simulink model "eCS_Old_Algo_And_Tests"  (R2015b)
settings: Solver=VariableStepAuto  StartTime=0.0  StopTime=10.0  RelTol=1e-3
values from neighbouring files (symbols this model uses):
  pulsetype = 2    [Parameter_eCS_Algo.m]    (also in run_simulation.m = j; run_simulation_ActiveX.m = j)
  rotation = 0    [Parameter_eCS_Algo.m]
  SubPulseType = 1    [Parameter_eCS_Algo.m]
undefined symbols (not defined in the file or in its folder): ddv, DiscIntNeverNeededParam, ECE_45_ax, ECE_45_ay, ECE_45_time, gmw_roada_x__m_s__, gmw_roada_y__m_s__, gmw_roadtime_2kHz, Heiko_AY, Heiko_AY_time, Meldorf_HindenburgstraAcceleration_x__m_s_2_, Meldorf_HindenburgstraAcceleration_y__m_s_2_, Meldorf_HindenburgstraTime__s_, pulse_FF27, pulse_MPDB, pulse_ODB40, pulse_ODB64, pulse_USNCAP, pulsetime_FF27, pulsetime_MPDB, pulsetime_ODB40, pulsetime_ODB64, pulsetime_USNCAP, VW_416_2kHza_x_2kHz, VW_416_2kHza_y_2kHz, VW_416_2kHztime_2kHz
libraries: tllib x9, simulink x9
(part 3 of 8)

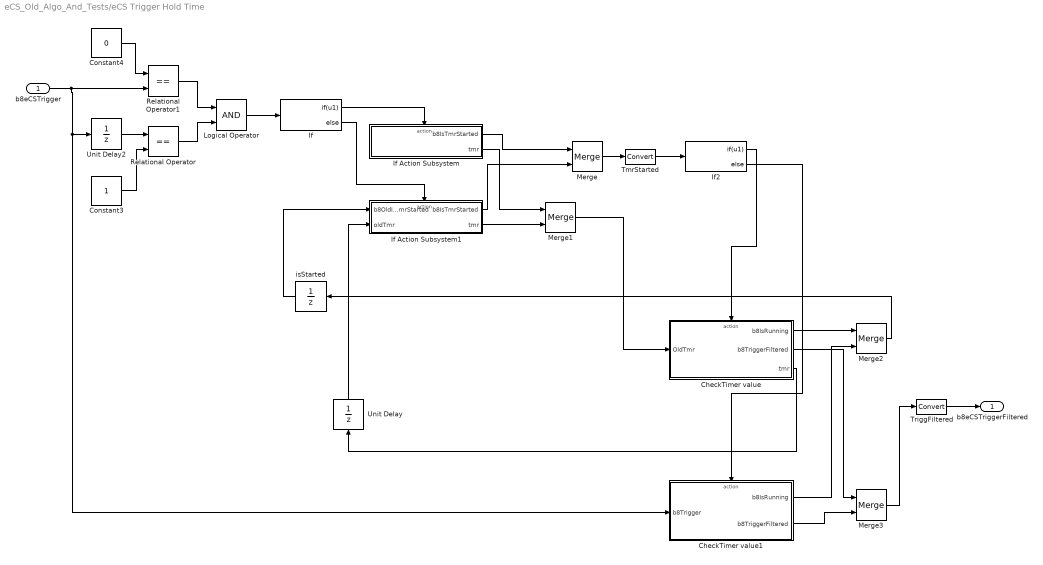
== system eCS_Old_Algo_And_Tests/eCS Trigger Hold Time ==
  b8eCSTrigger : Inport
  CheckTimer value : Subsystem  TreatAsAtomicUnit=on
  CheckTimer value1 : Subsystem  TreatAsAtomicUnit=on
  Constant3 : Constant  mask(TL_Constant){data={'date',738071.59305222228}}
      settings: CopyFcn=if exist('tl_reset_reviewflag') == 2, tl_reset_reviewflag(gcbh); end  DeleteFcn=if exist('delete_tlblock','file')==2,delete_tlblock(gcbh);end  NameChangeFcn=if exist('rename_tlblock','file')==2,rename_tlblock(gcbh);end  OpenFcn=if exist('tl_open_blockdlg','file')==2,tl_open_blockdlg(gcbh);else,open_system(gcbh,'parameter');end
      mask Help: eval(['if exist(''tl_online_help'',''file'') == 2, tl_online_help(''Topic'',''TL_Constant''),else, web([''jar:file:///'',matlabroot,''/help/toolbox/simulink/help.jar!/slref/' lower(get_param(gcbh,'Blocktype')) '.html''], ''-helpbrowser''),end'])
      mask Display: plot([-0.1, 1.05, NaN, -0.1, 1.05],[.01, .01, NaN, .99, .99]);
  Constant4 : Constant  Value=0  mask(TL_Constant){data={'date',738071.59305231483}}
      settings: CopyFcn=if exist('tl_reset_reviewflag') == 2, tl_reset_reviewflag(gcbh); end  DeleteFcn=if exist('delete_tlblock','file')==2,delete_tlblock(gcbh);end  NameChangeFcn=if exist('rename_tlblock','file')==2,rename_tlblock(gcbh);end  OpenFcn=if exist('tl_open_blockdlg','file')==2,tl_open_blockdlg(gcbh);else,open_system(gcbh,'parameter');end
      mask Help: eval(['if exist(''tl_online_help'',''file'') == 2, tl_online_help(''Topic'',''TL_Constant''),else, web([''jar:file:///'',matlabroot,''/help/toolbox/simulink/help.jar!/slref/' lower(get_param(gcbh,'Blocktype')) '.html''], ''-helpbrowser''),end'])
      mask Display: plot([-0.1, 1.05, NaN, -0.1, 1.05],[.01, .01, NaN, .99, .99]);
  If : If  IfExpression=u1
  If Action Subsystem : Subsystem  TreatAsAtomicUnit=on
  If Action Subsystem1 : Subsystem  TreatAsAtomicUnit=on
  If2 : If  IfExpression=u1
  Logical Operator : Logic  AllPortsSameDT=off  OutDataTypeStr=boolean  mask(TL_LogicalOperator){data={'date',738071.59305260412}}
      settings: DeleteFcn=if exist('delete_tlblock','file')==2,delete_tlblock(gcbh);end  NameChangeFcn=if exist('rename_tlblock','file')==2,rename_tlblock(gcbh);end  OpenFcn=if exist('tl_open_blockdlg','file')==2,tl_open_blockdlg(gcbh);else,open_system(gcbh,'parameter');end
      mask Help: eval(['if exist(''tl_online_help'',''file'') == 2, tl_online_help(''Topic'',''TL_LogicalOperator''),else, web([''jar:file:///'',matlabroot,''/help/toolbox/simulink/help.jar!/slref/' lower(get_param(gcbh,'Blocktype')) '.html''], ''-helpbrowser''),end'])
      mask Display: plot([-0.1, 1.05, NaN, -0.1, 1.05],[.01, .01, NaN, .99, .99]);
  Merge : Merge  InitialOutput=0  mask(TL_Merge){data={'date',738071.59305268514}}
      settings: CopyFcn=if exist('tl_reset_reviewflag') == 2, tl_reset_reviewflag(gcbh); end  DeleteFcn=if exist('delete_tlblock','file')==2,delete_tlblock(gcbh);end  NameChangeFcn=if exist('rename_tlblock','file')==2,rename_tlblock(gcbh);end  OpenFcn=if exist('tl_open_blockdlg','file')==2,tl_open_blockdlg(gcbh);else,open_system(gcbh,'parameter');end
      mask Help: eval(['if exist(''tl_online_help'',''file'') == 2, tl_online_help(''Topic'',''TL_Merge''),else, web([''jar:file:///'',matlabroot,''/help/toolbox/simulink/help.jar!/slref/' lower(get_param(gcbh,'Blocktype')) '.html''], ''-helpbrowser''),end'])
      mask Display: plot([-0.1, 1.05, NaN, -0.1, 1.05],[.01, .01, NaN, .99, .99]);
  Merge1 : Merge  InitialOutput=0  mask(TL_Merge){data={'date',738071.59305276617}}
      settings: CopyFcn=if exist('tl_reset_reviewflag') == 2, tl_reset_reviewflag(gcbh); end  DeleteFcn=if exist('delete_tlblock','file')==2,delete_tlblock(gcbh);end  NameChangeFcn=if exist('rename_tlblock','file')==2,rename_tlblock(gcbh);end  OpenFcn=if exist('tl_open_blockdlg','file')==2,tl_open_blockdlg(gcbh);else,open_system(gcbh,'parameter');end
      mask Help: eval(['if exist(''tl_online_help'',''file'') == 2, tl_online_help(''Topic'',''TL_Merge''),else, web([''jar:file:///'',matlabroot,''/help/toolbox/simulink/help.jar!/slref/' lower(get_param(gcbh,'Blocktype')) '.html''], ''-helpbrowser''),end'])
      mask Display: plot([-0.1, 1.05, NaN, -0.1, 1.05],[.01, .01, NaN, .99, .99]);
  Merge2 : Merge  InitialOutput=0  mask(TL_Merge){data={'date',738071.59305284719}}
      settings: CopyFcn=if exist('tl_reset_reviewflag') == 2, tl_reset_reviewflag(gcbh); end  DeleteFcn=if exist('delete_tlblock','file')==2,delete_tlblock(gcbh);end  NameChangeFcn=if exist('rename_tlblock','file')==2,rename_tlblock(gcbh);end  OpenFcn=if exist('tl_open_blockdlg','file')==2,tl_open_blockdlg(gcbh);else,open_system(gcbh,'parameter');end
      mask Help: eval(['if exist(''tl_online_help'',''file'') == 2, tl_online_help(''Topic'',''TL_Merge''),else, web([''jar:file:///'',matlabroot,''/help/toolbox/simulink/help.jar!/slref/' lower(get_param(gcbh,'Blocktype')) '.html''], ''-helpbrowser''),end'])
      mask Display: plot([-0.1, 1.05, NaN, -0.1, 1.05],[.01, .01, NaN, .99, .99]);
  Merge3 : Merge  InitialOutput=0  mask(TL_Merge){data={'date',738071.59305292822}}
      settings: CopyFcn=if exist('tl_reset_reviewflag') == 2, tl_reset_reviewflag(gcbh); end  DeleteFcn=if exist('delete_tlblock','file')==2,delete_tlblock(gcbh);end  NameChangeFcn=if exist('rename_tlblock','file')==2,rename_tlblock(gcbh);end  OpenFcn=if exist('tl_open_blockdlg','file')==2,tl_open_blockdlg(gcbh);else,open_system(gcbh,'parameter');end
      mask Help: eval(['if exist(''tl_online_help'',''file'') == 2, tl_online_help(''Topic'',''TL_Merge''),else, web([''jar:file:///'',matlabroot,''/help/toolbox/simulink/help.jar!/slref/' lower(get_param(gcbh,'Blocktype')) '.html''], ''-helpbrowser''),end'])
      mask Display: plot([-0.1, 1.05, NaN, -0.1, 1.05],[.01, .01, NaN, .99, .99]);
  Relational Operator : RelationalOperator  Operator===  OutDataTypeStr=boolean  mask(TL_RelationalOperator){data={'date',738071.59305300924}}
      settings: DeleteFcn=if exist('delete_tlblock','file')==2,delete_tlblock(gcbh);end  NameChangeFcn=if exist('rename_tlblock','file')==2,rename_tlblock(gcbh);end  OpenFcn=if exist('tl_open_blockdlg','file')==2,tl_open_blockdlg(gcbh);else,open_system(gcbh,'parameter');end
      mask Help: eval(['if exist(''tl_online_help'',''file'') == 2, tl_online_help(''Topic'',''TL_RelationalOperator''),else, web([''jar:file:///'',matlabroot,''/help/toolbox/simulink/help.jar!/slref/' lower(get_param(gcbh,'Blocktype')) '.html''], ''-helpbrowser''),end'])
      mask Display: plot([-0.1, 1.05, NaN, -0.1, 1.05],[.01, .01, NaN, .99, .99]);
  Relational Operator1 : RelationalOperator  Operator===  OutDataTypeStr=boolean  mask(TL_RelationalOperator){data={'date',738071.59305305558}}
      settings: DeleteFcn=if exist('delete_tlblock','file')==2,delete_tlblock(gcbh);end  NameChangeFcn=if exist('rename_tlblock','file')==2,rename_tlblock(gcbh);end  OpenFcn=if exist('tl_open_blockdlg','file')==2,tl_open_blockdlg(gcbh);else,open_system(gcbh,'parameter');end
      mask Help: eval(['if exist(''tl_online_help'',''file'') == 2, tl_online_help(''Topic'',''TL_RelationalOperator''),else, web([''jar:file:///'',matlabroot,''/help/toolbox/simulink/help.jar!/slref/' lower(get_param(gcbh,'Blocktype')) '.html''], ''-helpbrowser''),end'])
      mask Display: plot([-0.1, 1.05, NaN, -0.1, 1.05],[.01, .01, NaN, .99, .99]);
  TmrStarted : DataTypeConversion  mask(TL_Rescaler){data={'output',{'type','Bool'},'date',738071.59305305558}}
      settings: DeleteFcn=if exist('delete_tlblock','file')==2,delete_tlblock(gcbh);end  NameChangeFcn=if exist('rename_tlblock','file')==2,rename_tlblock(gcbh);end  OpenFcn=if exist('tl_open_blockdlg','file')==2,tl_open_blockdlg(gcbh);else,open_system(gcbh,'parameter');end
      mask Help: eval(['if exist(''tl_online_help'',''file'') == 2, tl_online_help(''Topic'',''TL_Rescaler''),else, web([''jar:file:///'',matlabroot,''/help/toolbox/simulink/help.jar!/slref/' lower(get_param(gcbh,'Blocktype')) '.html''], ''-helpbrowser''),end'])
      mask Display: plot([-0.1, 1.05, NaN, -0.1, 1.05],[.01, .01, NaN, .99, .99]);
  TriggFiltered : DataTypeConversion  mask(TL_Rescaler){data={'output',{'type','Bool'},'date',738073.43387922458}}
      settings: DeleteFcn=if exist('delete_tlblock','file')==2,delete_tlblock(gcbh);end  NameChangeFcn=if exist('rename_tlblock','file')==2,rename_tlblock(gcbh);end  OpenFcn=if exist('tl_open_blockdlg','file')==2,tl_open_blockdlg(gcbh);else,open_system(gcbh,'parameter');end
      mask Help: eval(['if exist(''tl_online_help'',''file'') == 2, tl_online_help(''Topic'',''TL_Rescaler''),else, web([''jar:file:///'',matlabroot,''/help/toolbox/simulink/help.jar!/slref/' lower(get_param(gcbh,'Blocktype')) '.html''], ''-helpbrowser''),end'])
      mask Display: plot([-0.1, 1.05, NaN, -0.1, 1.05],[.01, .01, NaN, .99, .99]);
  Unit Delay : UnitDelay  SampleTime=-1  mask(TL_UnitDelay){data={'output',{'type','UInt16'},'state',{'type','UInt16'},'date',738071.59305334487}}
      settings: CopyFcn=if exist('tl_reset_reviewflag') == 2, tl_reset_reviewflag(gcbh); end  DeleteFcn=if exist('delete_tlblock','file')==2,delete_tlblock(gcbh);end  NameChangeFcn=if exist('rename_tlblock','file')==2,rename_tlblock(gcbh);end  OpenFcn=if exist('tl_open_blockdlg','file')==2,tl_open_blockdlg(gcbh);else,open_system(gcbh,'parameter');end
      mask Help: eval(['if exist(''tl_online_help'',''file'') == 2, tl_online_help(''Topic'',''TL_UnitDelay''),else, web([''jar:file:///'',matlabroot,''/help/toolbox/simulink/help.jar!/slref/' lower(get_param(gcbh,'Blocktype')) '.html''], ''-helpbrowser''),end'])
      mask Display: plot([-0.1, 1.05, NaN, -0.1, 1.05],[.01, .01, NaN, .99, .99]);
  Unit Delay2 : UnitDelay  SampleTime=-1  mask(TL_UnitDelay){data={'output',{'type','UInt8'},'state',{'type','UInt8'},'date',738071.59305344906}}
      settings: CopyFcn=if exist('tl_reset_reviewflag') == 2, tl_reset_reviewflag(gcbh); end  DeleteFcn=if exist('delete_tlblock','file')==2,delete_tlblock(gcbh);end  NameChangeFcn=if exist('rename_tlblock','file')==2,rename_tlblock(gcbh);end  OpenFcn=if exist('tl_open_blockdlg','file')==2,tl_open_blockdlg(gcbh);else,open_system(gcbh,'parameter');end
      mask Help: eval(['if exist(''tl_online_help'',''file'') == 2, tl_online_help(''Topic'',''TL_UnitDelay''),else, web([''jar:file:///'',matlabroot,''/help/toolbox/simulink/help.jar!/slref/' lower(get_param(gcbh,'Blocktype')) '.html''], ''-helpbrowser''),end'])
      mask Display: plot([-0.1, 1.05, NaN, -0.1, 1.05],[.01, .01, NaN, .99, .99]);
  isStarted : UnitDelay  SampleTime=-1  mask(TL_UnitDelay){data={'output',{'type','Bool'},'state',{'type','Bool'},'date',738071.59305354161}}
      settings: CopyFcn=if exist('tl_reset_reviewflag') == 2, tl_reset_reviewflag(gcbh); end  DeleteFcn=if exist('delete_tlblock','file')==2,delete_tlblock(gcbh);end  NameChangeFcn=if exist('rename_tlblock','file')==2,rename_tlblock(gcbh);end  OpenFcn=if exist('tl_open_blockdlg','file')==2,tl_open_blockdlg(gcbh);else,open_system(gcbh,'parameter');end
      mask Help: eval(['if exist(''tl_online_help'',''file'') == 2, tl_online_help(''Topic'',''TL_UnitDelay''),else, web([''jar:file:///'',matlabroot,''/help/toolbox/simulink/help.jar!/slref/' lower(get_param(gcbh,'Blocktype')) '.html''], ''-helpbrowser''),end'])
      mask Display: plot([-0.1, 1.05, NaN, -0.1, 1.05],[.01, .01, NaN, .99, .99]);
  b8eCSTriggerFiltered : Outport
  wires:
  TmrStarted/1 -> If2/1
  Merge1/1 -> CheckTimer value/1(OldTmr)
  TriggFiltered/1 -> b8eCSTriggerFiltered/1
  Merge3/1 -> TriggFiltered/1
  CheckTimer value1/1(b8IsRunning) -> Merge2/2
  CheckTimer value/1(b8IsRunning) -> Merge2/1
  Merge2/1 -> isStarted/1
  If2/2 -> CheckTimer value1/Action
  Unit Delay/1 -> If Action Subsystem1/2(oldTmr)
  CheckTimer value/3(tmr) -> Unit Delay/1
  If Action Subsystem1/2(tmr) -> Merge1/2
  If Action Subsystem/2(tmr) -> Merge1/1
  isStarted/1 -> If Action Subsystem1/1(b8OldIsTmrStarted)
  Merge/1 -> TmrStarted/1
  If Action Subsystem1/1(b8IsTmrStarted) -> Merge/2
  If Action Subsystem/1(b8IsTmrStarted) -> Merge/1
  If/2 -> If Action Subsystem1/Action
  Relational Operator/1 -> Logical Operator/2
  Relational Operator1/1 -> Logical Operator/1
  Logical Operator/1 -> If/1
  Constant4/1 -> Relational Operator1/1
  Constant3/1 -> Relational Operator/2
  Unit Delay2/1 -> Relational Operator/1
  b8eCSTrigger/1 -> Unit Delay2/1, CheckTimer value1/1(b8Trigger), Relational Operator1/2
  If2/1 -> CheckTimer value/Action
  If/1 -> If Action Subsystem/Action
  CheckTimer value1/2(b8TriggerFiltered) -> Merge3/2
  CheckTimer value/2(b8TriggerFiltered) -> Merge3/1

== system eCS_Old_Algo_And_Tests/eCS_Algo_in_g ==
  Ax (g) : Inport  PortDimensions=1
  Ay (g) : Inport  Port=2  PortDimensions=1
  Action Port : ActionPort
  Ax dual integrator : Subsystem  TreatAsAtomicUnit=on
  Ay dual integrator : Subsystem  TreatAsAtomicUnit=on
  Crash Acceleration : Subsystem  TreatAsAtomicUnit=on
  Gain : Gain  Gain=ddv('gSecSquareToMM')  mask(TL_Gain){data={'output',{'type','UInt16','lsb',2^-14,'unit','m'},'gain',{'variable','gSecSquareToMM'},'date',737951.40928561345}}
      settings: CopyFcn=if exist('tl_reset_reviewflag') == 2, tl_reset_reviewflag(gcbh); end  DeleteFcn=if exist('delete_tlblock','file')==2,delete_tlblock(gcbh);end  NameChangeFcn=if exist('rename_tlblock','file')==2,rename_tlblock(gcbh);end  OpenFcn=if exist('tl_open_blockdlg','file')==2,tl_open_blockdlg(gcbh);else,open_system(gcbh,'parameter');end
      mask Help: eval(['if exist(''tl_online_help'',''file'') == 2, tl_online_help(''Topic'',''TL_Gain''),else, web([''jar:file:///'',matlabroot,''/help/toolbox/simulink/help.jar!/slref/' lower(get_param(gcbh,'Blocktype')) '.html''], ''-helpbrowser''),end'])
      mask Display: plot([0, .88, 0],[.05, .5, .93]);
  Vector Norm : Subsystem  TreatAsAtomicUnit=on
  eCS Trigger Hold Time : Subsystem  TreatAsAtomicUnit=on
  mergedTrigger : Logic  Operator=OR  AllPortsSameDT=off  OutDataTypeStr=boolean  mask(TL_LogicalOperator){data={'date',737961.51872327551}}
      settings: DeleteFcn=if exist('delete_tlblock','file')==2,delete_tlblock(gcbh);end  NameChangeFcn=if exist('rename_tlblock','file')==2,rename_tlblock(gcbh);end  OpenFcn=if exist('tl_open_blockdlg','file')==2,tl_open_blockdlg(gcbh);else,open_system(gcbh,'parameter');end
      mask Help: eval(['if exist(''tl_online_help'',''file'') == 2, tl_online_help(''Topic'',''TL_LogicalOperator''),else, web([''jar:file:///'',matlabroot,''/help/toolbox/simulink/help.jar!/slref/' lower(get_param(gcbh,'Blocktype')) '.html''], ''-helpbrowser''),end'])
      mask Display: plot([-0.1, 1.05, NaN, -0.1, 1.05],[.01, .01, NaN, .99, .99]);
  s_ball : Outport
  eCSTrigger : Outport  Port=2
  wires:
  Gain/1 -> s_ball/1
  Ay dual integrator/1(Sy (g.s²)) -> Vector Norm/2(Sy)
  Crash Acceleration/1(b8CrashTrigger) -> mergedTrigger/2
  Ax dual integrator/1(Sx (g.s²)) -> Vector Norm/1(Sx)
  Ay (g)/1 -> Ay dual integrator/1(Ay (g)), Crash Acceleration/2(Ay)
  eCS Trigger Hold Time/1(b8eCSTriggerFiltered) -> eCSTrigger/1
  Vector Norm/1(s_ball) -> Gain/1
  Ax (g)/1 -> Crash Acceleration/1(Ax), Ax dual integrator/1(Ax (g))
  Vector Norm/2(b8PositionTrigger) -> mergedTrigger/1
  mergedTrigger/1 -> eCS Trigger Hold Time/1(b8eCSTrigger)

== system eCS_Old_Algo_And_Tests/eCS_Algo_in_g1 ==
  Ax (g) : Inport  PortDimensions=1
  Ay (g) : Inport  Port=2  PortDimensions=1
  Action Port : ActionPort
  Ax dual integrator : Subsystem  TreatAsAtomicUnit=on
  Ay dual integrator : Subsystem  TreatAsAtomicUnit=on
  Crash Acceleration : Subsystem  TreatAsAtomicUnit=on
  Gain : Gain  Gain=ddv('gSecSquareToMM')  mask(TL_Gain){data={'output',{'type','UInt16','lsb',2^-14,'unit','m'},'gain',{'variable','gSecSquareToMM'},'date',737951.40928561345}}
      settings: CopyFcn=if exist('tl_reset_reviewflag') == 2, tl_reset_reviewflag(gcbh); end  DeleteFcn=if exist('delete_tlblock','file')==2,delete_tlblock(gcbh);end  NameChangeFcn=if exist('rename_tlblock','file')==2,rename_tlblock(gcbh);end  OpenFcn=if exist('tl_open_blockdlg','file')==2,tl_open_blockdlg(gcbh);else,open_system(gcbh,'parameter');end
      mask Help: eval(['if exist(''tl_online_help'',''file'') == 2, tl_online_help(''Topic'',''TL_Gain''),else, web([''jar:file:///'',matlabroot,''/help/toolbox/simulink/help.jar!/slref/' lower(get_param(gcbh,'Blocktype')) '.html''], ''-helpbrowser''),end'])
      mask Display: plot([0, .88, 0],[.05, .5, .93]);
  Vector Norm : Subsystem  TreatAsAtomicUnit=on
  eCS Trigger Hold Time : Subsystem  TreatAsAtomicUnit=on
  mergedTrigger : Logic  Operator=OR  AllPortsSameDT=off  OutDataTypeStr=boolean  mask(TL_LogicalOperator){data={'date',737961.51872327551}}
      settings: DeleteFcn=if exist('delete_tlblock','file')==2,delete_tlblock(gcbh);end  NameChangeFcn=if exist('rename_tlblock','file')==2,rename_tlblock(gcbh);end  OpenFcn=if exist('tl_open_blockdlg','file')==2,tl_open_blockdlg(gcbh);else,open_system(gcbh,'parameter');end
      mask Help: eval(['if exist(''tl_online_help'',''file'') == 2, tl_online_help(''Topic'',''TL_LogicalOperator''),else, web([''jar:file:///'',matlabroot,''/help/toolbox/simulink/help.jar!/slref/' lower(get_param(gcbh,'Blocktype')) '.html''], ''-helpbrowser''),end'])
      mask Display: plot([-0.1, 1.05, NaN, -0.1, 1.05],[.01, .01, NaN, .99, .99]);
  s_ball : Outport
  eCSTrigger : Outport  Port=2
  wires:
  Gain/1 -> s_ball/1
  Ay dual integrator/1(Sy (g.s²)) -> Vector Norm/2(Sy)
  Crash Acceleration/1(b8CrashTrigger) -> mergedTrigger/2
  Ax dual integrator/1(Sx (g.s²)) -> Vector Norm/1(Sx)
  Ay (g)/1 -> Ay dual integrator/1(Ay (g)), Crash Acceleration/2(Ay)
  eCS Trigger Hold Time/1(b8eCSTriggerFiltered) -> eCSTrigger/1
  Vector Norm/1(s_ball) -> Gain/1
  Ax (g)/1 -> Crash Acceleration/1(Ax), Ax dual integrator/1(Ax (g))
  Vector Norm/2(b8PositionTrigger) -> mergedTrigger/1
  mergedTrigger/1 -> eCS Trigger Hold Time/1(b8eCSTrigger)

== system eCS_Old_Algo_And_Tests/eCS_norm_algo ==
  note: Ball Algo
  Ax (m.s-2) : Inport
  Ay (m.s-2) : Inport  Port=2
  Action Port : ActionPort
  Ax dual integrator : Subsystem  TreatAsAtomicUnit=on
  Vector Norm : Subsystem  TreatAsAtomicUnit=on
  eCS Trigger Hold Time : Subsystem  TreatAsAtomicUnit=on
  mToMm : Gain  Gain=ddv('MToMM')  mask(TL_Gain){data={'output',{'type','UInt16','lsb',2^-14,'unit','m'},'gain',{'variable','MToMM'},'date',737954.64461454866}}
      settings: CopyFcn=if exist('tl_reset_reviewflag') == 2, tl_reset_reviewflag(gcbh); end  DeleteFcn=if exist('delete_tlblock','file')==2,delete_tlblock(gcbh);end  NameChangeFcn=if exist('rename_tlblock','file')==2,rename_tlblock(gcbh);end  OpenFcn=if exist('tl_open_blockdlg','file')==2,tl_open_blockdlg(gcbh);else,open_system(gcbh,'parameter');end
      mask Help: eval(['if exist(''tl_online_help'',''file'') == 2, tl_online_help(''Topic'',''TL_Gain''),else, web([''jar:file:///'',matlabroot,''/help/toolbox/simulink/help.jar!/slref/' lower(get_param(gcbh,'Blocktype')) '.html''], ''-helpbrowser''),end'])
      mask Display: plot([0, .88, 0],[.05, .5, .93]);
  s_ball : Outport
  eCSTrigger : Outport  Port=2
  wires:
  Ay (m.s-2)/1 -> Vector Norm/2(Ay)
  Ax dual integrator/2(eCSTrigger) -> eCS Trigger Hold Time/1(b8eCSTrigger)
  mToMm/1 -> s_ball/1
  eCS Trigger Hold Time/1(b8eCSTriggerFiltered) -> eCSTrigger/1
  Ax (m.s-2)/1 -> Vector Norm/1(Ax)
  Vector Norm/1(Accel) -> Ax dual integrator/1(Ax (m.s-2))
  Ax dual integrator/1(Sx (m)) -> mToMm/1

== system eCS_Old_Algo_And_Tests/Input (Pulse// Angle)_OLD/Puls_GWM_road_C.Morgan ==
  time in : Inport
  Constant : Constant  Value=gmw_roadtime_2kHz
  Constant1 : Constant  Value=gmw_roada_x__m_s__
  Constant3 : Constant  Value=gmw_roada_y__m_s__
  Lookup Table Dynamic : simulink/Lookup Tables/Lookup Table Dynamic  LookUpMeth=Interpolation-Use End Values  OutDataTypeStr=fixdt('double')  OutputDataTypeScalingMode=Specify via dialog  OutDataType=fixdt('double')  OutScaling=[]  DoSatur=off
  Lookup Table Dynamic1 : simulink/Lookup Tables/Lookup Table Dynamic  LookUpMeth=Interpolation-Use End Values  OutDataTypeStr=fixdt('double')  OutputDataTypeScalingMode=Specify via dialog  OutDataType=fixdt('double')  OutScaling=[]  DoSatur=off
  Mux : Mux  Inputs=2
  Rate Transition1 : RateTransition
  Rate Transition2 : RateTransition  OutPortSampleTime=1/2000
  Scope : Scope
  m/s² to g : Gain  Gain=1/9.81
  pulse out [x,y] (g) : Outport
  wires:
  Mux/1 -> m/s² to g/1
  m/s² to g/1 -> Rate Transition1/1
  Rate Transition1/1 -> pulse out [x,y] (g)/1, Scope/1
  Constant3/1 -> Lookup Table Dynamic1/3
  Constant/1 -> Lookup Table Dynamic/2, Lookup Table Dynamic1/2
  Constant1/1 -> Lookup Table Dynamic/3
  time in/1 -> Rate Transition2/1
  Lookup Table Dynamic1/1 -> Mux/2
  Rate Transition2/1 -> Lookup Table Dynamic/1, Lookup Table Dynamic1/1
  Lookup Table Dynamic/1 -> Mux/1

== system eCS_Old_Algo_And_Tests/Input (Pulse// Angle)_OLD/Puls_Kopfsteinpflaster Meldorf Hindenburgstrasse ==
  time in : Inport
  Constant : Constant  Value=Meldorf_HindenburgstraTime__s_
  Constant1 : Constant  Value=Meldorf_HindenburgstraAcceleration_x__m_s_2_
  Constant3 : Constant  Value=Meldorf_HindenburgstraAcceleration_y__m_s_2_
  Lookup Table Dynamic : simulink/Lookup Tables/Lookup Table Dynamic  LookUpMeth=Interpolation-Use End Values  OutDataTypeStr=fixdt('double')  OutputDataTypeScalingMode=Specify via dialog  OutDataType=fixdt('double')  OutScaling=[]  DoSatur=off
  Lookup Table Dynamic1 : simulink/Lookup Tables/Lookup Table Dynamic  LookUpMeth=Interpolation-Use End Values  OutDataTypeStr=fixdt('double')  OutputDataTypeScalingMode=Specify via dialog  OutDataType=fixdt('double')  OutScaling=[]  DoSatur=off
  Mux : Mux  Inputs=2
  Rate Transition1 : RateTransition
  Rate Transition2 : RateTransition  OutPortSampleTime=1/500
  Scope : Scope
  m/s² to g : Gain  Gain=1/9.81
  pulse out [x,y] (g) : Outport
  wires:
  Lookup Table Dynamic/1 -> Mux/1
  Rate Transition2/1 -> Lookup Table Dynamic1/1, Lookup Table Dynamic/1
  Lookup Table Dynamic1/1 -> Mux/2
  time in/1 -> Rate Transition2/1
  Constant1/1 -> Lookup Table Dynamic/3
  Constant/1 -> Lookup Table Dynamic1/2, Lookup Table Dynamic/2
  Constant3/1 -> Lookup Table Dynamic1/3
  Rate Transition1/1 -> Scope/1, pulse out [x,y] (g)/1
  m/s² to g/1 -> Rate Transition1/1
  Mux/1 -> m/s² to g/1

== system eCS_Old_Algo_And_Tests/Input (Pulse// Angle)_OLD/Puls_VW416_Atlas_C.Morgan ==
  time in : Inport
  Constant : Constant  Value=VW_416_2kHztime_2kHz
  Constant1 : Constant  Value=VW_416_2kHza_x_2kHz
  Constant3 : Constant  Value=VW_416_2kHza_y_2kHz
  Lookup Table Dynamic : simulink/Lookup Tables/Lookup Table Dynamic  LookUpMeth=Interpolation-Use End Values  OutDataTypeStr=fixdt('double')  OutputDataTypeScalingMode=Specify via dialog  OutDataType=fixdt('double')  OutScaling=[]  DoSatur=off
  Lookup Table Dynamic1 : simulink/Lookup Tables/Lookup Table Dynamic  LookUpMeth=Interpolation-Use End Values  OutDataTypeStr=fixdt('double')  OutputDataTypeScalingMode=Specify via dialog  OutDataType=fixdt('double')  OutScaling=[]  DoSatur=off
  Mux : Mux  Inputs=2
  Rate Transition1 : RateTransition
  Rate Transition2 : RateTransition  OutPortSampleTime=1/2000
  Scope : Scope
  pulse out [x,y] (g) : Outport
  wires:
  Mux/1 -> Rate Transition1/1
  Rate Transition1/1 -> pulse out [x,y] (g)/1, Scope/1
  Constant3/1 -> Lookup Table Dynamic1/3
  Constant/1 -> Lookup Table Dynamic/2, Lookup Table Dynamic1/2
  Constant1/1 -> Lookup Table Dynamic/3
  time in/1 -> Rate Transition2/1
  Lookup Table Dynamic1/1 -> Mux/2
  Rate Transition2/1 -> Lookup Table Dynamic/1, Lookup Table Dynamic1/1
  Lookup Table Dynamic/1 -> Mux/1

== system eCS_Old_Algo_And_Tests/Input (Pulse// Angle)_OLD/Rotation ==
  Generic_Pulse : Inport
  Constant : Constant  Value=-90
  Gain : Gain  Gain=pi/180
  Gain1 : Gain  Gain=pi/180
  Product : Product
  Product1 : Product
  Subtract : Sum  Inputs=+-
  Trigonometric Function : Trigonometry  Operator=cos
  Trigonometric Function1 : Trigonometry  Operator=cos
  sled rotation : Constant  Value=rotation
  ax_rot : Outport
  ay_rot : Outport  Port=2
  wires:
  Trigonometric Function/1 -> Product/1
  Trigonometric Function1/1 -> Product1/1
  sled rotation/1 -> Subtract/2, Gain/1
  Gain1/1 -> Trigonometric Function1/1
  Gain/1 -> Trigonometric Function/1
  Constant/1 -> Subtract/1
  Subtract/1 -> Gain1/1
  Generic_Pulse/1 -> Product1/2, Product/2
  Product/1 -> ax_rot/1
  Product1/1 -> ay_rot/1

== system eCS_Old_Algo_And_Tests/Input (Pulse// Angle)_OLD/Triggered Subsystem ==
  Trigger : TriggerPort
  Add : Sum
  Constant : Constant  Value=2^-14
  Delay : Delay  DelayLength=1  InitialCondition=0
  Scope : Scope
  Out1 : Outport
  wires:
  Add/1 -> Delay/1, Scope/1, Out1/1
  Constant/1 -> Add/2
  Delay/1 -> Add/1

== system eCS_Old_Algo_And_Tests/eCS Trigger Hold Time/CheckTimer value ==
  OldTmr : Inport
  Action Port : ActionPort
  Constant : Constant  mask(TL_Constant){data={'date',738071.59305151622}}
      settings: CopyFcn=if exist('tl_reset_reviewflag') == 2, tl_reset_reviewflag(gcbh); end  DeleteFcn=if exist('delete_tlblock','file')==2,delete_tlblock(gcbh);end  NameChangeFcn=if exist('rename_tlblock','file')==2,rename_tlblock(gcbh);end  OpenFcn=if exist('tl_open_blockdlg','file')==2,tl_open_blockdlg(gcbh);else,open_system(gcbh,'parameter');end
      mask Help: eval(['if exist(''tl_online_help'',''file'') == 2, tl_online_help(''Topic'',''TL_Constant''),else, web([''jar:file:///'',matlabroot,''/help/toolbox/simulink/help.jar!/slref/' lower(get_param(gcbh,'Blocktype')) '.html''], ''-helpbrowser''),end'])
      mask Display: plot([-0.1, 1.05, NaN, -0.1, 1.05],[.01, .01, NaN, .99, .99]);
  Constant1 : Constant  Value=0  mask(TL_Constant){data={'date',738071.59305159724}}
      settings: CopyFcn=if exist('tl_reset_reviewflag') == 2, tl_reset_reviewflag(gcbh); end  DeleteFcn=if exist('delete_tlblock','file')==2,delete_tlblock(gcbh);end  NameChangeFcn=if exist('rename_tlblock','file')==2,rename_tlblock(gcbh);end  OpenFcn=if exist('tl_open_blockdlg','file')==2,tl_open_blockdlg(gcbh);else,open_system(gcbh,'parameter');end
      mask Help: eval(['if exist(''tl_online_help'',''file'') == 2, tl_online_help(''Topic'',''TL_Constant''),else, web([''jar:file:///'',matlabroot,''/help/toolbox/simulink/help.jar!/slref/' lower(get_param(gcbh,'Blocktype')) '.html''], ''-helpbrowser''),end'])
      mask Display: plot([-0.1, 1.05, NaN, -0.1, 1.05],[.01, .01, NaN, .99, .99]);
  Constant2 : Constant  mask(TL_Constant){data={'date',738071.59305167827}}
      settings: CopyFcn=if exist('tl_reset_reviewflag') == 2, tl_reset_reviewflag(gcbh); end  DeleteFcn=if exist('delete_tlblock','file')==2,delete_tlblock(gcbh);end  NameChangeFcn=if exist('rename_tlblock','file')==2,rename_tlblock(gcbh);end  OpenFcn=if exist('tl_open_blockdlg','file')==2,tl_open_blockdlg(gcbh);else,open_system(gcbh,'parameter');end
      mask Help: eval(['if exist(''tl_online_help'',''file'') == 2, tl_online_help(''Topic'',''TL_Constant''),else, web([''jar:file:///'',matlabroot,''/help/toolbox/simulink/help.jar!/slref/' lower(get_param(gcbh,'Blocktype')) '.html''], ''-helpbrowser''),end'])
      mask Display: plot([-0.1, 1.05, NaN, -0.1, 1.05],[.01, .01, NaN, .99, .99]);
  Constant3 : Constant  mask(TL_Constant){data={'date',738071.59305175929}}
      settings: CopyFcn=if exist('tl_reset_reviewflag') == 2, tl_reset_reviewflag(gcbh); end  DeleteFcn=if exist('delete_tlblock','file')==2,delete_tlblock(gcbh);end  NameChangeFcn=if exist('rename_tlblock','file')==2,rename_tlblock(gcbh);end  OpenFcn=if exist('tl_open_blockdlg','file')==2,tl_open_blockdlg(gcbh);else,open_system(gcbh,'parameter');end
      mask Help: eval(['if exist(''tl_online_help'',''file'') == 2, tl_online_help(''Topic'',''TL_Constant''),else, web([''jar:file:///'',matlabroot,''/help/toolbox/simulink/help.jar!/slref/' lower(get_param(gcbh,'Blocktype')) '.html''], ''-helpbrowser''),end'])
      mask Display: plot([-0.1, 1.05, NaN, -0.1, 1.05],[.01, .01, NaN, .99, .99]);
  Rescaler : DataTypeConversion  mask(TL_Rescaler){data={'output',{'type','Bool'},'date',738071.59305184032}}
      settings: DeleteFcn=if exist('delete_tlblock','file')==2,delete_tlblock(gcbh);end  NameChangeFcn=if exist('rename_tlblock','file')==2,rename_tlblock(gcbh);end  OpenFcn=if exist('tl_open_blockdlg','file')==2,tl_open_blockdlg(gcbh);else,open_system(gcbh,'parameter');end
      mask Help: eval(['if exist(''tl_online_help'',''file'') == 2, tl_online_help(''Topic'',''TL_Rescaler''),else, web([''jar:file:///'',matlabroot,''/help/toolbox/simulink/help.jar!/slref/' lower(get_param(gcbh,'Blocktype')) '.html''], ''-helpbrowser''),end'])
      mask Display: plot([-0.1, 1.05, NaN, -0.1, 1.05],[.01, .01, NaN, .99, .99]);
  RollingCntr : Sum  mask(TL_Sum){data={'output',{'type','UInt16'},'date',738071.5930519097}}
      settings: CopyFcn=if exist('tl_reset_reviewflag') == 2, tl_reset_reviewflag(gcbh); end  DeleteFcn=if exist('delete_tlblock','file')==2,delete_tlblock(gcbh);end  NameChangeFcn=if exist('rename_tlblock','file')==2,rename_tlblock(gcbh);end  OpenFcn=if exist('tl_open_blockdlg','file')==2,tl_open_blockdlg(gcbh);else,open_system(gcbh,'parameter');end
      mask Help: eval(['if exist(''tl_online_help'',''file'') == 2, tl_online_help(''Topic'',''TL_Sum''),else, web([''jar:file:///'',matlabroot,''/help/toolbox/simulink/help.jar!/slref/' lower(get_param(gcbh,'Blocktype')) '.html''], ''-helpbrowser''),end'])
      mask Display: plot([-0.1, 1.05, NaN, -0.1, 1.05],[.01, .01, NaN, .99, .99]);
  Switch : Switch  Threshold=ddv('eCS_CFG/ECS_HOLDING_TRIGGER')  mask(TL_Switch){data={'output',{'type','Bool'},'threshold',{'variable','eCS_CFG/ECS_HOLDING_TRIGGER'},'date',738071.59305200237}}
      settings: CopyFcn=if exist('tl_reset_reviewflag') == 2, tl_reset_reviewflag(gcbh); end  DeleteFcn=if exist('delete_tlblock','file')==2,delete_tlblock(gcbh);end  NameChangeFcn=if exist('rename_tlblock','file')==2,rename_tlblock(gcbh);end  OpenFcn=if exist('tl_open_blockdlg','file')==2,tl_open_blockdlg(gcbh);else,open_system(gcbh,'parameter');end
      mask Help: eval(['if exist(''tl_online_help'',''file'') == 2, tl_online_help(''Topic'',''TL_Switch''),else, web([''jar:file:///'',matlabroot,''/help/toolbox/simulink/help.jar!/slref/' lower(get_param(gcbh,'Blocktype')) '.html''], ''-helpbrowser''),end'])
      mask Display: plot([-0.1, 1.05, NaN, -0.1, 1.05],[.01, .01, NaN, .99, .99]);
  b8IsRunning : Outport  InitialOutput=0
  b8TriggerFiltered : Outport  Port=2  InitialOutput=0
  tmr : Outport  Port=3  InitialOutput=0
  wires:
  Rescaler/1 -> b8TriggerFiltered/1
  OldTmr/1 -> RollingCntr/2
  Constant3/1 -> Rescaler/1
  Constant2/1 -> Switch/3
  Constant1/1 -> Switch/1
  Constant/1 -> RollingCntr/1
  RollingCntr/1 -> Switch/2, tmr/1
  Switch/1 -> b8IsRunning/1

== system eCS_Old_Algo_And_Tests/eCS Trigger Hold Time/CheckTimer value1 ==
  b8Trigger : Inport
  Action Port : ActionPort
  Constant1 : Constant  Value=0  mask(TL_Constant){data={'date',738071.59305214125}}
      settings: CopyFcn=if exist('tl_reset_reviewflag') == 2, tl_reset_reviewflag(gcbh); end  DeleteFcn=if exist('delete_tlblock','file')==2,delete_tlblock(gcbh);end  NameChangeFcn=if exist('rename_tlblock','file')==2,rename_tlblock(gcbh);end  OpenFcn=if exist('tl_open_blockdlg','file')==2,tl_open_blockdlg(gcbh);else,open_system(gcbh,'parameter');end
      mask Help: eval(['if exist(''tl_online_help'',''file'') == 2, tl_online_help(''Topic'',''TL_Constant''),else, web([''jar:file:///'',matlabroot,''/help/toolbox/simulink/help.jar!/slref/' lower(get_param(gcbh,'Blocktype')) '.html''], ''-helpbrowser''),end'])
      mask Display: plot([-0.1, 1.05, NaN, -0.1, 1.05],[.01, .01, NaN, .99, .99]);
  b8IsRunning : Outport  InitialOutput=0
  b8TriggerFiltered : Outport  Port=2  InitialOutput=0
  wires:
  Constant1/1 -> b8IsRunning/1
  b8Trigger/1 -> b8TriggerFiltered/1

== system eCS_Old_Algo_And_Tests/eCS Trigger Hold Time/If Action Subsystem ==
  Action Port : ActionPort
  Constant : Constant  mask(TL_Constant){data={'date',738071.59305240738}}
      settings: CopyFcn=if exist('tl_reset_reviewflag') == 2, tl_reset_reviewflag(gcbh); end  DeleteFcn=if exist('delete_tlblock','file')==2,delete_tlblock(gcbh);end  NameChangeFcn=if exist('rename_tlblock','file')==2,rename_tlblock(gcbh);end  OpenFcn=if exist('tl_open_blockdlg','file')==2,tl_open_blockdlg(gcbh);else,open_system(gcbh,'parameter');end
      mask Help: eval(['if exist(''tl_online_help'',''file'') == 2, tl_online_help(''Topic'',''TL_Constant''),else, web([''jar:file:///'',matlabroot,''/help/toolbox/simulink/help.jar!/slref/' lower(get_param(gcbh,'Blocktype')) '.html''], ''-helpbrowser''),end'])
      mask Display: plot([-0.1, 1.05, NaN, -0.1, 1.05],[.01, .01, NaN, .99, .99]);
  Constant1 : Constant  Value=0  mask(TL_Constant){data={'date',738071.5930524884}}
      settings: CopyFcn=if exist('tl_reset_reviewflag') == 2, tl_reset_reviewflag(gcbh); end  DeleteFcn=if exist('delete_tlblock','file')==2,delete_tlblock(gcbh);end  NameChangeFcn=if exist('rename_tlblock','file')==2,rename_tlblock(gcbh);end  OpenFcn=if exist('tl_open_blockdlg','file')==2,tl_open_blockdlg(gcbh);else,open_system(gcbh,'parameter');end
      mask Help: eval(['if exist(''tl_online_help'',''file'') == 2, tl_online_help(''Topic'',''TL_Constant''),else, web([''jar:file:///'',matlabroot,''/help/toolbox/simulink/help.jar!/slref/' lower(get_param(gcbh,'Blocktype')) '.html''], ''-helpbrowser''),end'])
      mask Display: plot([-0.1, 1.05, NaN, -0.1, 1.05],[.01, .01, NaN, .99, .99]);
  b8IsTmrStarted : Outport  InitialOutput=0
  tmr : Outport  Port=2  InitialOutput=0
  wires:
  Constant1/1 -> tmr/1
  Constant/1 -> b8IsTmrStarted/1

== system eCS_Old_Algo_And_Tests/eCS Trigger Hold Time/If Action Subsystem1 ==
  b8OldIsTmrStarted : Inport
  oldTmr : Inport  Port=2
  Action Port : ActionPort
  b8IsTmrStarted : Outport  InitialOutput=0
  tmr : Outport  Port=2  InitialOutput=0
  wires:
  oldTmr/1 -> tmr/1
  b8OldIsTmrStarted/1 -> b8IsTmrStarted/1

== system eCS_Old_Algo_And_Tests/eCS_Algo_in_g/Ax dual integrator ==
  note: sc: 1e-4
  note: sc: 1e-3
  note: sc: 1e-3
  note: sc: 1e-3
  note: x-axis : 1e-8
      | y-axis : 1e-4
      | output : 1e-4
  note: sc: 1e-6
  note: [-1 : 1]
  note: [-2 ; +2] g
      | [-32768 ; 32767] LSB
  note: Sat [-0.0001 ; 0.0001]g.s²
      | [-10000;10000] LSB
      | scaling : 1e-8
  note: [0 ; 25]
  note: [0 ;25]
  note: [-2; 2]g => [-32768 ; +32767] LSB
      | scaling : 2^-14
  note: sc: 1e-6
  Ax (g) : Inport
  AddAngle : Sum  mask(TL_Sum){data={'output',{'scaling','PowerOf2/scAngle'},'date',737951.68910436344}}
      settings: CopyFcn=if exist('tl_reset_reviewflag','file')==2,tl_reset_reviewflag(gcbh);end  DeleteFcn=if exist('delete_tlblock','file')==2,delete_tlblock(gcbh);end  NameChangeFcn=if exist('rename_tlblock','file')==2,rename_tlblock(gcbh);end  OpenFcn=if exist('tl_open_blockdlg','file')==2,tl_open_blockdlg(gcbh);else,open_system(gcbh,'parameter');end
      mask Help: eval(['if exist(''tl_online_help'',''file'') == 2, tl_online_help(''Topic'',''TL_Sum''),else, web([''jar:file:///'',matlabroot,''/help/toolbox/simulink/help.jar!/slref/' lower(get_param(gcbh,'Blocktype')) '.html''], ''-helpbrowser''),end'])
      mask Display: plot([-0.1, 1.05, NaN, -0.1, 1.05],[.01, .01, NaN, .99, .99]);
  AddAx : Sum  Inputs=+--  mask(TL_Sum){data={'output',{'type','Int32','scaling','PowerOf2/scIntegV'},'date',737961.51711288199}}
      settings: CopyFcn=if exist('tl_reset_reviewflag','file')==2,tl_reset_reviewflag(gcbh);end  DeleteFcn=if exist('delete_tlblock','file')==2,delete_tlblock(gcbh);end  NameChangeFcn=if exist('rename_tlblock','file')==2,rename_tlblock(gcbh);end  OpenFcn=if exist('tl_open_blockdlg','file')==2,tl_open_blockdlg(gcbh);else,open_system(gcbh,'parameter');end
      mask Help: eval(['if exist(''tl_online_help'',''file'') == 2, tl_online_help(''Topic'',''TL_Sum''),else, web([''jar:file:///'',matlabroot,''/help/toolbox/simulink/help.jar!/slref/' lower(get_param(gcbh,'Blocktype')) '.html''], ''-helpbrowser''),end'])
      mask Display: plot([-0.1, 1.05, NaN, -0.1, 1.05],[.01, .01, NaN, .99, .99]);
  AxCalotteAngle1 : Gain  Gain=ddv('eCS_CFG/g_algo/S16_CALOTTE_ANGLE_1')  mask(TL_Gain){data={'output',{'scaling','PowerOf2/scAngle'},'gain',{'variable','eCS_CFG/g_algo/S16_CALOTTE_ANGLE_1'},'date',737958.36049306719}}
      settings: CopyFcn=if exist('tl_reset_reviewflag','file')==2,tl_reset_reviewflag(gcbh);end  DeleteFcn=if exist('delete_tlblock','file')==2,delete_tlblock(gcbh);end  NameChangeFcn=if exist('rename_tlblock','file')==2,rename_tlblock(gcbh);end  OpenFcn=if exist('tl_open_blockdlg','file')==2,tl_open_blockdlg(gcbh);else,open_system(gcbh,'parameter');end
      mask Help: eval(['if exist(''tl_online_help'',''file'') == 2, tl_online_help(''Topic'',''TL_Gain''),else, web([''jar:file:///'',matlabroot,''/help/toolbox/simulink/help.jar!/slref/' lower(get_param(gcbh,'Blocktype')) '.html''], ''-helpbrowser''),end'])
      mask Display: plot([0, .88, 0],[.05, .5, .93]);
  AxCalotteAngle2 : Gain  Gain=ddv('eCS_CFG/g_algo/S16_CALOTTE_ANGLE_2')  mask(TL_Gain){data={'output',{'scaling','PowerOf2/scAngle'},'gain',{'variable','eCS_CFG/g_algo/S16_CALOTTE_ANGLE_2'},'date',737958.36059362267}}
      settings: CopyFcn=if exist('tl_reset_reviewflag','file')==2,tl_reset_reviewflag(gcbh);end  DeleteFcn=if exist('delete_tlblock','file')==2,delete_tlblock(gcbh);end  NameChangeFcn=if exist('rename_tlblock','file')==2,rename_tlblock(gcbh);end  OpenFcn=if exist('tl_open_blockdlg','file')==2,tl_open_blockdlg(gcbh);else,open_system(gcbh,'parameter');end
      mask Help: eval(['if exist(''tl_online_help'',''file'') == 2, tl_online_help(''Topic'',''TL_Gain''),else, web([''jar:file:///'',matlabroot,''/help/toolbox/simulink/help.jar!/slref/' lower(get_param(gcbh,'Blocktype')) '.html''], ''-helpbrowser''),end'])
      mask Display: plot([0, .88, 0],[.05, .5, .93]);
  BallDamperSat : Saturate  UpperLimit=ddv('eCS_CFG/g_algo/BALL_DAMPER_SAT_MAX')  LowerLimit=ddv('eCS_CFG/g_algo/BALL_DAMPER_SAT_MIN')  mask(TL_Saturate){data={'output',{'type','Int32','scaling','PowerOf2/scIntegV'},'lowerlimit',{'variable','eCS_CFG/g_algo/BALL_DAMPER_SAT_MIN'},'upperlimit',{'variable','eCS_CFG/g_algo/BALL_DAMPER_SAT_MAX'},'date',737957.666285382}}
      settings: CopyFcn=if exist('tl_reset_reviewflag','file')==2,tl_reset_reviewflag(gcbh);end  DeleteFcn=if exist('delete_tlblock','file')==2,delete_tlblock(gcbh);end  NameChangeFcn=if exist('rename_tlblock','file')==2,rename_tlblock(gcbh);end  OpenFcn=if exist('tl_open_blockdlg','file')==2,tl_open_blockdlg(gcbh);else,open_system(gcbh,'parameter');end
      mask Help: eval(['if exist(''tl_online_help'',''file'') == 2, tl_online_help(''Topic'',''TL_Saturate''),else, web([''jar:file:///'',matlabroot,''/help/toolbox/simulink/help.jar!/slref/' lower(get_param(gcbh,'Blocktype')) '.html''], ''-helpbrowser''),end'])
      mask Display: plot([-0.1, 1.05, NaN, -0.1, 1.05],[.01, .01, NaN, .99, .99]);
  Function : tllib/Function  data={'stepfunctionname','ComputeSx','date',737937.64870774304}  displayString=FUNCTION
  IntegSx : DiscreteIntegrator  SampleTime=-1  LimitOutput=on  UpperSaturationLimit=ddv('eCS_CFG/g_algo/BALL_POS_MAX')  LowerSaturationLimit=ddv('eCS_CFG/g_algo/BALL_POS_MIN')  ICPrevOutput=DiscIntNeverNeededParam  ICPrevScaledInput=DiscIntNeverNeededParam  mask(TL_DiscreteIntegrator){data={'output',{'scaling','PowerOf2/scIntegS'},'state',{'scaling','PowerOf2/scIntegS'},'lowerlimit',{'variable','eCS_CFG/g_algo/BALL_POS_MIN'},'upperlimit',{'variable','eCS_CFG/g_algo/BALL_POS_MAX'},'date',737961.51726134261}}
      settings: CopyFcn=if exist('tl_reset_reviewflag') == 2, tl_reset_reviewflag(gcbh); end  DeleteFcn=if exist('delete_tlblock','file')==2,delete_tlblock(gcbh);end  NameChangeFcn=if exist('rename_tlblock','file')==2,rename_tlblock(gcbh);end  OpenFcn=if exist('tl_open_blockdlg','file')==2,tl_open_blockdlg(gcbh);else,open_system(gcbh,'parameter');end
      mask Help: eval(['if exist(''tl_online_help'',''file'') == 2, tl_online_help(''Topic'',''TL_DiscreteIntegrator''),else, web([''jar:file:///'',matlabroot,''/help/toolbox/simulink/help.jar!/slref/' lower(get_param(gcbh,'Blocktype')) '.html''], ''-helpbrowser''),end'])
      mask Display: plot([-0.1, 1.05, NaN, -0.1, 1.05],[.01, .01, NaN, .99, .99]);
  IntegVx : DiscreteIntegrator  SampleTime=-1  ICPrevOutput=DiscIntNeverNeededParam  ICPrevScaledInput=DiscIntNeverNeededParam  mask(TL_DiscreteIntegrator){data={'output',{'scaling','PowerOf2/scIntegV'},'state',{'scaling','PowerOf2/scIntegV'},'date',737961.51719508099}}
      settings: CopyFcn=if exist('tl_reset_reviewflag') == 2, tl_reset_reviewflag(gcbh); end  DeleteFcn=if exist('delete_tlblock','file')==2,delete_tlblock(gcbh);end  NameChangeFcn=if exist('rename_tlblock','file')==2,rename_tlblock(gcbh);end  OpenFcn=if exist('tl_open_blockdlg','file')==2,tl_open_blockdlg(gcbh);else,open_system(gcbh,'parameter');end
      mask Help: eval(['if exist(''tl_online_help'',''file'') == 2, tl_online_help(''Topic'',''TL_DiscreteIntegrator''),else, web([''jar:file:///'',matlabroot,''/help/toolbox/simulink/help.jar!/slref/' lower(get_param(gcbh,'Blocktype')) '.html''], ''-helpbrowser''),end'])
      mask Display: plot([-0.1, 1.05, NaN, -0.1, 1.05],[.01, .01, NaN, .99, .99]);
  Scope1 : Scope
  SinAx : Trigonometry  mask(TL_Trigonometry){data={'output',{'scaling','PowerOf2/scRadian'},'date',737961.51746089116}}
      settings: CopyFcn=if exist('tl_reset_reviewflag','file')==2,tl_reset_reviewflag(gcbh);end  DeleteFcn=if exist('delete_tlblock','file')==2,delete_tlblock(gcbh);end  NameChangeFcn=if exist('rename_tlblock','file')==2,rename_tlblock(gcbh);end  OpenFcn=if exist('tl_open_blockdlg','file')==2,tl_open_blockdlg(gcbh);else,open_system(gcbh,'parameter');end
      mask Help: eval(['if exist(''tl_online_help'',''file'') == 2, tl_online_help(''Topic'',''TL_Trigonometry''),else, web([''jar:file:///'',matlabroot,''/help/toolbox/simulink/help.jar!/slref/' lower(get_param(gcbh,'Blocktype')) '.html''], ''-helpbrowser''),end'])
      mask Display: plot([-0.1, 1.05, NaN, -0.1, 1.05],[.01, .01, NaN, .99, .99]);
  ball damper : Gain  Gain=ddv('eCS_CFG/g_algo/BALL_DAMPER_COEFF')  mask(TL_Gain){data={'output',{'type','Int32','scaling','PowerOf2/scIntegV'},'gain',{'variable','eCS_CFG/g_algo/BALL_DAMPER_COEFF'},'date',737954.47214212967}}
      settings: CopyFcn=if exist('tl_reset_reviewflag','file')==2,tl_reset_reviewflag(gcbh);end  DeleteFcn=if exist('delete_tlblock','file')==2,delete_tlblock(gcbh);end  NameChangeFcn=if exist('rename_tlblock','file')==2,rename_tlblock(gcbh);end  OpenFcn=if exist('tl_open_blockdlg','file')==2,tl_open_blockdlg(gcbh);else,open_system(gcbh,'parameter');end
      mask Help: eval(['if exist(''tl_online_help'',''file'') == 2, tl_online_help(''Topic'',''TL_Gain''),else, web([''jar:file:///'',matlabroot,''/help/toolbox/simulink/help.jar!/slref/' lower(get_param(gcbh,'Blocktype')) '.html''], ''-helpbrowser''),end'])
      mask Display: plot([0, .88, 0],[.05, .5, .93]);
  grad in rad1 : Gain  Gain=pi/180  mask(TL_Gain){data={'output',{'scaling','PowerOf2/scLutY'},'date',737951.6866806366}}
      settings: CopyFcn=if exist('tl_reset_reviewflag','file')==2,tl_reset_reviewflag(gcbh);end  DeleteFcn=if exist('delete_tlblock','file')==2,delete_tlblock(gcbh);end  NameChangeFcn=if exist('rename_tlblock','file')==2,rename_tlblock(gcbh);end  OpenFcn=if exist('tl_open_blockdlg','file')==2,tl_open_blockdlg(gcbh);else,open_system(gcbh,'parameter');end
      mask Help: eval(['if exist(''tl_online_help'',''file'') == 2, tl_online_help(''Topic'',''TL_Gain''),else, web([''jar:file:///'',matlabroot,''/help/toolbox/simulink/help.jar!/slref/' lower(get_param(gcbh,'Blocktype')) '.html''], ''-helpbrowser''),end'])
      mask Display: plot([0, .88, 0],[.05, .5, .93]);
  soft sign1 : Lookup_n-D  NumberOfTableDimensions=1  BreakpointsForDimension1=ddv('eCS_CFG/g_algo/AS8LUT_CALLOTE_ANGLE_1_IDX')  IndexSearchMethod=Linear search  Table=ddv('eCS_CFG/g_algo/AS32LUT_CALLOTE_ANGLE_1_FACT')  ExtrapMethod=Clip  UseLastTableValue=on  InternalRulePriority=Speed  RndMeth=Simplest  InputSameDT=on  mask(TL_Lookup1D){data={'input',{'variable','eCS_CFG/g_algo/AS8LUT_CALLOTE_ANGLE_1_IDX'},'output',{'scaling','PowerOf2/scLutY'},'table',{'variable','eCS_CFG/g_algo/AS32LUT_CALLOTE_ANGLE_1_FACT'},'map',{'name','gCalotteAngle1_LUT','class','MERGEABLE_CONST'},'date',738070.37874855322}}
      settings: CopyFcn=if exist('tl_reset_reviewflag','file')==2,tl_reset_reviewflag(gcbh);end  DeleteFcn=if exist('delete_tlblock','file')==2,delete_tlblock(gcbh);end  NameChangeFcn=if exist('rename_tlblock','file')==2,rename_tlblock(gcbh);end  OpenFcn=if exist('tl_open_blockdlg','file')==2,tl_open_blockdlg(gcbh);else,open_system(gcbh,'parameter');end
      mask Help: eval(['if exist(''tl_online_help'',''file'') == 2, tl_online_help(''Topic'',''TL_Lookup1D''),else, web([''jar:file:///'',matlabroot,''/help/toolbox/simulink/help.jar!/slref/' lower(get_param(gcbh,'Blocktype')) '.html''], ''-helpbrowser''),end'])
      mask Display: plot([-0.1, 1.05, NaN, -0.1, 1.05],[.01, .01, NaN, .99, .99]);
  soft sign2 : Lookup_n-D  NumberOfTableDimensions=1  BreakpointsForDimension1=ddv('eCS_CFG/g_algo/LUT_CALLOTE_ANGLE_2_IDX')  IndexSearchMethod=Linear search  Table=ddv('eCS_CFG/g_algo/LUT_CALLOTE_ANGLE_2_FACT')  ExtrapMethod=Clip  UseLastTableValue=on  InternalRulePriority=Speed  RndMeth=Simplest  InputSameDT=on  mask(TL_Lookup1D){data={'input',{'variable','eCS_CFG/g_algo/LUT_CALLOTE_ANGLE_2_IDX'},'output',{'scaling','PowerOf2/scLutY'},'table',{'variable','eCS_CFG/g_algo/LUT_CALLOTE_ANGLE_2_FACT'},'map',{'name','gCalotteAngle2_LUT','class','MERGEABLE_CONST'},'date',738070.37884137733}}
      settings: CopyFcn=if exist('tl_reset_reviewflag','file')==2,tl_reset_reviewflag(gcbh);end  DeleteFcn=if exist('delete_tlblock','file')==2,delete_tlblock(gcbh);end  NameChangeFcn=if exist('rename_tlblock','file')==2,rename_tlblock(gcbh);end  OpenFcn=if exist('tl_open_blockdlg','file')==2,tl_open_blockdlg(gcbh);else,open_system(gcbh,'parameter');end
      mask Help: eval(['if exist(''tl_online_help'',''file'') == 2, tl_online_help(''Topic'',''TL_Lookup1D''),else, web([''jar:file:///'',matlabroot,''/help/toolbox/simulink/help.jar!/slref/' lower(get_param(gcbh,'Blocktype')) '.html''], ''-helpbrowser''),end'])
      mask Display: plot([-0.1, 1.05, NaN, -0.1, 1.05],[.01, .01, NaN, .99, .99]);
  Sx (g.s²) : Outport
  wires:
  AddAx/1 -> IntegVx/1, Scope1/1  "a-ref"
  Ax (g)/1 -> AddAx/1
  IntegVx/1 -> ball damper/1, IntegSx/1
  SinAx/1 -> AddAx/2
  BallDamperSat/1 -> AddAx/3
  grad in rad1/1 -> SinAx/1
  soft sign1/1 -> AxCalotteAngle1/1
  AxCalotteAngle1/1 -> AddAngle/1
  soft sign2/1 -> AxCalotteAngle2/1
  AxCalotteAngle2/1 -> AddAngle/2
  AddAngle/1 -> grad in rad1/1
  ball damper/1 -> BallDamperSat/1
  IntegSx/1 -> soft sign2/1, soft sign1/1, Sx (g.s²)/1
